simulink model "block_2ndorder"  (R2017b)
settings: Solver=VariableStepAuto  StartTime=0.0  StopTime=10.0  RelTol=1e-3
settings Model: Creator=Nick  LastModifiedBy=Nick

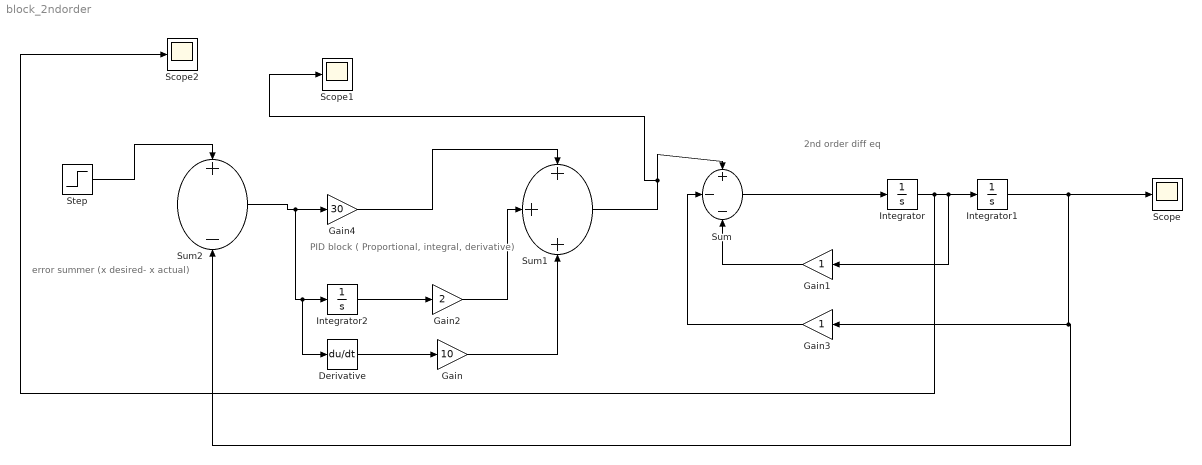
== system block_2ndorder ==
  note: 2nd order diff eq
  note: PID block ( Proportional, integral, derivative)
  note: error summer (x desired- x actual)
  Derivative : Derivative
  Gain : Gain  Gain=10
  Gain1 : Gain
  Gain2 : Gain  Gain=2
  Gain3 : Gain
  Gain4 : Gain  Gain=30
  Integrator : Integrator
  Integrator1 : Integrator
  Integrator2 : Integrator
  Scope : Scope
  Scope1 : Scope
  Scope2 : Scope
  Step : Step  Time=2  SampleTime=0
  Sum : Sum  Inputs=+--
  Sum1 : Sum  Inputs=+++
  Sum2 : Sum  Inputs=+-
  wires:
  Integrator/1 -> Scope2/1, Gain1/1, Integrator1/1
  Integrator1/1 -> Sum2/2, Gain3/1, Scope/1
  Sum/1 -> Integrator/1
  Gain3/1 -> Sum/2
  Gain1/1 -> Sum/3
  Integrator2/1 -> Gain2/1
  Derivative/1 -> Gain/1
  Gain2/1 -> Sum1/2
  Gain/1 -> Sum1/3
  Gain4/1 -> Sum1/1
  Sum1/1 -> Scope1/1, Sum/1
  Sum2/1 -> Derivative/1, Integrator2/1, Gain4/1
  Step/1 -> Sum2/1
